simulink model "Oakland_Mission_Server"  (R2019a)
settings: Solver=ode4  StartTime=0.0  StopTime=inf  FixedStep=1/1000  RelTol=1e-3  EnableMultiTasking=on
model workspace (MAT data in the model file):
  cameraStepSize = Simulink.Parameter
  cameraStepSize.Value = Simulink.data.Expression
  cameraStepSize.Value.ExpressionString = "qc_get_step_size * ceil (1/30 /qc_get_step_size)"
  cameraStepSize.DataType = 'auto'
  cameraStepSize.Dimensions = -1
  mainStepSize = Simulink.Parameter
  mainStepSize.Value = Simulink.data.Expression
  mainStepSize.Value.ExpressionString = "qc_get_step_size"
  mainStepSize.DataType = 'auto'
  mainStepSize.Dimensions = -1
libraries: quarc_library x7
settings Model: SimulationMode=external  ExtModeTrigDuration=10000  OrderedModelArguments=off  Creator=mbohra  LastModifiedBy=Derek
settings SolverCC: PositivePriorityOrder=on
settings DataIOCC: ReturnWorkspaceOutputs=off
settings DebuggingCC: ArithmeticOperatorsInVariantConditions=warning
settings SFSimCC: SimUseLocalCustomCode=off
settings RTWCC: SystemTargetFile=quarc_win64.tlc  TemplateMakefile=quarc_default_tmf  Description=QUARC Win64 Target Using Toolchain  RTWUseLocalCustomCode=off  Toolchain=QUARC win64 | nmake (64-bit Windows)  BuildConfiguration=Faster Runs
settings CodeAppCC: StateflowObjectComments=on
settings STFCustomTargetCC: TargetLangStandard=C99 (ISO)  ConcurrentExecutionCompliant=on  UseToolchainInfoCompliant=on  SystemTargetFile=quarc_win64.tlc
settings GRTTargetCC: ParMdlRefBuildCompliant=off  CompOptLevelCompliant=off  CombineOutputUpdateFcns=off  MatFileLogging=off  CPPClassGenCompliant=off  GRTInterface=on  ExtMode=on  ExtModeMexFile=quarc_comm
settings ConfigComp: CovMetricSettings=dswe

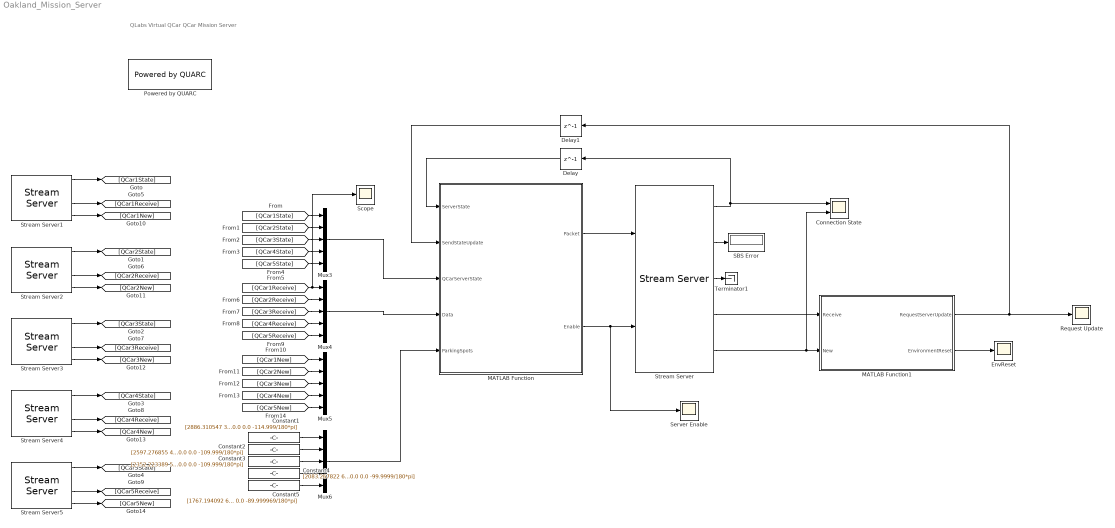
== system Oakland_Mission_Server ==
  note: QLabs Virtual QCar
      | QCar Mission Server
  "Connection State " : Scope  NumInputPorts=2
  Constant1 : Constant  Value=[2886.310547 365.284058 20.712402 0.0 0.0 -114.999/180*pi]
  Constant2 : Constant  Value=[2597.276855 484.31073 20.712402 0.0 0.0 -109.999/180*pi]
  Constant3 : Constant  Value=[2352.223389 588.301392 20.712524 0.0 0.0 -109.999/180*pi]
  Constant4 : Constant  Value=[2083.267822 660.12085 20.712402 0.0 0.0 -99.9999/180*pi]
  Constant5 : Constant  Value=[1767.194092 667.67334 20.713074 0.0 0.0 -89.999969/180*pi]
  Delay : Delay  DelayLength=1
  Delay1 : Delay  DelayLength=1
  "EnvReset " : Scope
  MATLAB Function : MATLAB Function  TreatAsAtomicUnit=on
  MATLAB Function1 : MATLAB Function  TreatAsAtomicUnit=on
  Mux{3..6} (4 alike) : Mux  Inputs=5
  Powered by QUARC : quarc_library/Logos/Powered by QUARC
  Request Update : Scope
  SBS Error : Display
  Scope : Scope
  Server Enable : Scope
  Stream Server : quarc_library/Communications/Basic/Stream Server  uri_source=Specify via dialog (do not evaluate)  uri=tcpip://remotehost:18001?nagle='off'  apply_uri_to_all_configs=on  send_buffer_size=65537  receive_buffer_size=65537  byte_order=little endian (Intel - LSB first)  optimization=Minimum latency  send_options=Send all data  receive_options=Receive all data  default_value=[0]  sample_time=qc_get_step_size  active=on  implementation=Use blocking I/O in a separate thread  send_fifo_size=3  receive_fifo_size=3  send_priority=0  receive_priority=0  send_dimensions=on  receive_dimensions=on  max_dimensions=65537  data_type=uint8  type_expr=BusObject
      settings: AttributesFormatString="\"tcpip://remotehost:18001?nagle='off'\""
  Stream Server1 : quarc_library/Communications/Basic/Stream Server  uri_source=Specify via dialog (do not evaluate)  uri=tcpip://remotehost:18005?nagle='off'  apply_uri_to_all_configs=on  send_buffer_size=1460  receive_buffer_size=1460  byte_order=little endian (Intel - LSB first)  optimization=Minimum latency  send_options=Do not send data  receive_options=Receive all data  default_value=[0 0 0 0 0 0]  sample_time=qc_get_step_size  active=off  implementation=Use blocking I/O in a separate thread  send_fifo_size=3  receive_fifo_size=3  send_priority=0  receive_priority=0  send_dimensions=off  receive_dimensions=off  max_dimensions=-1  data_type=single  type_expr=BusObject
      settings: AttributesFormatString="\"tcpip://remotehost:18005?nagle='off'\""
  Stream Server2 : quarc_library/Communications/Basic/Stream Server  uri_source=Specify via dialog (do not evaluate)  uri=tcpip://remotehost:18006?nagle='off'  apply_uri_to_all_configs=on  send_buffer_size=1460  receive_buffer_size=1460  byte_order=little endian (Intel - LSB first)  optimization=Minimum latency  send_options=Do not send data  receive_options=Receive all data  default_value=[0 0 0 0 0 0]  sample_time=qc_get_step_size  active=off  implementation=Use blocking I/O in a separate thread  send_fifo_size=3  receive_fifo_size=3  send_priority=0  receive_priority=0  send_dimensions=off  receive_dimensions=off  max_dimensions=-1  data_type=single  type_expr=BusObject
      settings: AttributesFormatString="\"tcpip://remotehost:18006?nagle='off'\""
  Stream Server3 : quarc_library/Communications/Basic/Stream Server  uri_source=Specify via dialog (do not evaluate)  uri=tcpip://remotehost:18007?nagle='off'  apply_uri_to_all_configs=on  send_buffer_size=1460  receive_buffer_size=1460  byte_order=little endian (Intel - LSB first)  optimization=Minimum latency  send_options=Do not send data  receive_options=Receive all data  default_value=[0 0 0 0 0 0]  sample_time=qc_get_step_size  active=off  implementation=Use blocking I/O in a separate thread  send_fifo_size=3  receive_fifo_size=3  send_priority=0  receive_priority=0  send_dimensions=off  receive_dimensions=off  max_dimensions=-1  data_type=single  type_expr=BusObject
      settings: AttributesFormatString="\"tcpip://remotehost:18007?nagle='off'\""
  Stream Server4 : quarc_library/Communications/Basic/Stream Server  uri_source=Specify via dialog (do not evaluate)  uri=tcpip://remotehost:18008?nagle='off'  apply_uri_to_all_configs=on  send_buffer_size=1460  receive_buffer_size=1460  byte_order=little endian (Intel - LSB first)  optimization=Minimum latency  send_options=Do not send data  receive_options=Receive all data  default_value=[0 0 0 0 0 0]  sample_time=qc_get_step_size  active=off  implementation=Use blocking I/O in a separate thread  send_fifo_size=3  receive_fifo_size=3  send_priority=0  receive_priority=0  send_dimensions=off  receive_dimensions=off  max_dimensions=-1  data_type=single  type_expr=BusObject
      settings: AttributesFormatString="\"tcpip://remotehost:18008?nagle='off'\""
  Stream Server5 : quarc_library/Communications/Basic/Stream Server  uri_source=Specify via dialog (do not evaluate)  uri=tcpip://remotehost:18009?nagle='off'  apply_uri_to_all_configs=on  send_buffer_size=1460  receive_buffer_size=1460  byte_order=little endian (Intel - LSB first)  optimization=Minimum latency  send_options=Do not send data  receive_options=Receive all data  default_value=[0 0 0 0 0 0]  sample_time=qc_get_step_size  active=off  implementation=Use blocking I/O in a separate thread  send_fifo_size=3  receive_fifo_size=3  send_priority=0  receive_priority=0  send_dimensions=off  receive_dimensions=off  max_dimensions=-1  data_type=single  type_expr=BusObject
      settings: AttributesFormatString="\"tcpip://remotehost:18009?nagle='off'\""
  Terminator1 : Terminator
  wires:
  Stream Server/3 -> Terminator1/1
  MATLAB Function/1(Packet) -> Stream Server/1
  MATLAB Function1/1(RequestServerUpdate) -> Request Update/1, Delay1/1
  Delay/1 -> MATLAB Function/1(ServerState)
  Delay1/1 -> MATLAB Function/2(SendStateUpdate)
  Stream Server/4 -> MATLAB Function1/1(Receive)
  MATLAB Function/2(Enable) -> Server Enable/1, Stream Server/2
  Stream Server/5 -> "Connection State "/2, MATLAB Function1/2(New)
  Stream Server/2 -> SBS Error/1
  Stream Server/1 -> Delay/1, "Connection State "/1
  Stream Server1/1 -> [QCar1State]
  Stream Server5/1 -> [QCar5State]
  Stream Server4/1 -> [QCar4State]
  Stream Server3/1 -> [QCar3State]
  Stream Server2/1 -> [QCar2State]
  Stream Server1/3 -> [QCar1Receive]
  Stream Server1/4 -> [QCar1New]
  Stream Server2/3 -> [QCar2Receive]
  Stream Server2/4 -> [QCar2New]
  Stream Server3/3 -> [QCar3Receive]
  Stream Server3/4 -> [QCar3New]
  Stream Server4/3 -> [QCar4Receive]
  Stream Server4/4 -> [QCar4New]
  Stream Server5/3 -> [QCar5Receive]
  Stream Server5/4 -> [QCar5New]
  [QCar1State] -> Mux3/1
  [QCar5State] -> Mux3/5
  [QCar4State] -> Mux3/4
  [QCar3State] -> Mux3/3
  [QCar2State] -> Mux3/2
  [QCar2Receive] -> Mux4/2
  [QCar3Receive] -> Mux4/3
  [QCar4Receive] -> Mux4/4
  [QCar5Receive] -> Mux4/5
  [QCar1Receive] -> Scope/1, Mux4/1
  [QCar2New] -> Mux5/2
  [QCar3New] -> Mux5/3
  [QCar4New] -> Mux5/4
  [QCar5New] -> Mux5/5
  [QCar1New] -> Mux5/1
  Mux3/1 -> MATLAB Function/3(QCarServerState)
  Mux4/1 -> MATLAB Function/4(Data)
  Constant1/1 -> Mux6/1
  Constant2/1 -> Mux6/2
  Constant5/1 -> Mux6/5
  Constant4/1 -> Mux6/4
  Constant3/1 -> Mux6/3
  Mux6/1 -> MATLAB Function/5(ParkingSpots)
  MATLAB Function1/2(EnvironmentReset) -> "EnvReset "/1

== matlab function Oakland_Mission_Server/MATLAB Function ==
  settings: updateMethod=DISCRETE  sampleTime=qc_get_step_size
  data: Packet output size=65537; ServerState input; SendStateUpdate input; Enable output; QCarServerState input; Data input; ParkingSpots input
function [Packet,Enable] = MakePacket(ServerState, SendStateUpdate, QCarServerState, Data, ParkingSpots) 

% Be sure to set the maximum signal size of the variable size Packet port 
% in Simulink->Edit Data of the editor window.  Size should be 65537 or
% larger to ensure that the stream server generates a 4 byte packet size.

%% Setup
persistent LastServerState;

if isempty(LastServerState)
    LastServerState = uint8(0);
end

Enable = 0;
Packet = uint8([]);


%% On connection
if ((ServerState == 2) && (LastServerState ~= 2))
    SendStateUpdate = uint8(1);
end

%%Normal operation

for i = 1:5

    %% Send new State Container
    % Previous state processed, send a new one
    if (SendStateUpdate)
        if (QCarServerState(i) == 2) 
            Packet = [Packet; QCarMakeSetTransformContainer(i, [(Data((i-1)*6+1)) (Data((i-1)*6+2)) (Data((i-1)*6+3))], [(Data((i-1)*6+4)) (Data((i-1)*6+5)) (Data((i-1)*6+6))], 0, 0, 0, 0, 0, 0)];
        else
            Packet = [Packet; QCarMakeSetTransformContainer(i, [(ParkingSpots((i-1)*6+1)) (ParkingSpots((i-1)*6+2)) (ParkingSpots((i-1)*6+3))], [(ParkingSpots((i-1)*6+4)) (ParkingSpots((i-1)*6+5)) (ParkingSpots((i-1)*6+6))], 0, 0, 0, 0, 0, 0)];
        end
    end

end

%% Transmit
% If we have data to send, enable the transmit
PacketLength = length(Packet);

if (PacketLength > 0)
    % Add magic byte.  This is just for error handling and isn't typically
    % required in simulink, but useful in lower-level languages like Python
    Packet = [uint8(123); Packet];
    
    Enable = 1; 
end

LastServerState = ServerState;

== matlab function Oakland_Mission_Server/MATLAB Function1 ==
  data: Receive input size=65537; RequestServerUpdate output; New input; EnvironmentReset output
function [RequestServerUpdate, EnvironmentReset] = DecodePacket(Receive, New)

%% Setup


% Need to assign outputs here even though they are reassigned at the end
% since matlab can't determine the signal widths
EnvironmentReset = 0;

RequestServerUpdate =  uint8(0);
PacketSize = length(Receive);

% Packet > 0, new data, and magic number in first index
if ((PacketSize > 0) && (New == 1) && (Receive(1) == uint8(123)))
    
    %skip magic number
    Index = int32(2);
    
    while(Index <= PacketSize)
       
        %% Get container details
        ContainerSize = typecast(uint8(flip(Receive(Index:Index+3))), 'int32');
        DeviceID = typecast(uint8(flip(Receive(Index+4:Index+7))), 'int32');
        DeviceNum = uint8(Receive(Index+8));
        DeviceFunction = uint8(Receive(Index+9));
        PayloadStart = Index+10;
        PayloadEnd = Index+ContainerSize-1;
        
        %% Pass container to appropriate decoding function
        if (DeviceID == 160) %is this a QCar container?
            
            if (DeviceFunction == 13) %UE4 State Response
                RequestServerUpdate = uint8(1);
            end
        
        elseif (DeviceID == 1001) %Simulink notification
            if (DeviceFunction == 200) %Reset button
                EnvironmentReset = 1;
            end
        end
        
        
        
        %% Process next container if any data is left.
        Index = Index+ContainerSize;
    end


end
